simulink model "Fct_app"  (R2018b)
settings: Solver=ode15s  StartTime=0.0  StopTime=T_s  MaxStep=1/(100*fn)  MinStep=1/(1000*fn)  RelTol=1e-3
values from neighbouring files (symbols this model uses):
  f = (alpha/100)*Pn/(Wn)^2    (= 0.000141076783904)    [MAS_EVV_init.m]    (also in fct_trans.m)
  Imr = phi_rd_n/Msr    [MAS_EVV_init.m]    (also in fct_trans.m)
  J = 0.51    [MAS_EVV_init.m]    (also in fct_trans.m)
  k_couple = 1/(0.3*sigma*Ts)    [MAS_EVV_init.m]    (also in fct_trans.m)
  k_omega = 1/(0.3*0.5)    (= 6.66666666667)    [MAS_EVV_init.m]    (also in fct_trans.m)
  k_phi = 1/(0.3*Tr)    [MAS_EVV_init.m]    (also in fct_trans.m)
  Lr = (N2w/2+L1w)/wn    [MAS_EVV_init.m]    (also in fct_trans.m)
  Msr = L1w/wn    [MAS_EVV_init.m]    (also in fct_trans.m)
  P = 1    [MAS_EVV_init.m]    (also in fct_trans.m)
  Rs = 0.9*Rr    [MAS_EVV_init.m]    (also in fct_trans.m)
  sigma = 1-(Msr^2)/(Ls*Lr)    [MAS_EVV_init.m]    (also in fct_trans.m)
  T_C_BF = 0.0445    [MAS_EVV_init.m]    (also in fct_trans.m)
  T_phi_BF = 0.3*Tr    [MAS_EVV_init.m]    (also in fct_trans.m)
  Tr = Lr/Rr    [MAS_EVV_init.m]    (also in fct_trans.m)
  Ts = Ls/Rs    [MAS_EVV_init.m]    (also in fct_trans.m)
  zero_couple = zero(C_couple)    [MAS_EVV_init.m]    (also in fct_trans.m)
  zero_omega = zero(C_omega)    [MAS_EVV_init.m]    (also in fct_trans.m)
  zero_phi = zero(C_phi)    [MAS_EVV_init.m]    (also in fct_trans.m)
undefined symbols (not defined in the file or in its folder): kcouple, komega, kphi
settings Model: Creator=cindyiskandar  LastModifiedBy=cindyiskandar

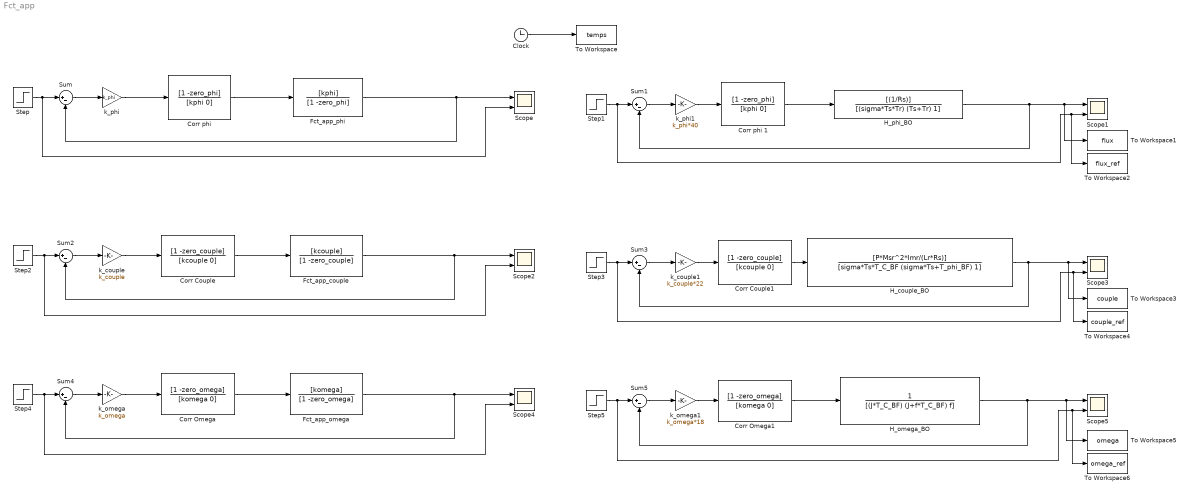
== system Fct_app ==
  Clock : Clock
  Corr Couple : TransferFcn  Numerator=[1 -zero_couple]  Denominator=[kcouple 0]
  Corr Couple1 : TransferFcn  Numerator=[1 -zero_couple]  Denominator=[kcouple 0]
  Corr Omega : TransferFcn  Numerator=[1 -zero_omega]  Denominator=[komega 0]
  Corr Omega1 : TransferFcn  Numerator=[1 -zero_omega]  Denominator=[komega 0]
  "Corr phi " : TransferFcn  Numerator=[1 -zero_phi]  Denominator=[kphi 0]
  Corr phi 1 : TransferFcn  Numerator=[1 -zero_phi]  Denominator=[kphi 0]
  Fct_app_couple : TransferFcn  Numerator=[kcouple]  Denominator=[1 -zero_couple]
  Fct_app_omega : TransferFcn  Numerator=[komega]  Denominator=[1 -zero_omega]
  "Fct_app_phi " : TransferFcn  Numerator=[kphi]  Denominator=[1 -zero_phi]
  H_couple_BO : TransferFcn  Numerator=[P*Msr^2*Imr/(Lr*Rs)]  Denominator=[sigma*Ts*T_C_BF (sigma*Ts+T_phi_BF) 1]
  H_omega_BO : TransferFcn  Denominator=[(J*T_C_BF) (J+f*T_C_BF) f]
  H_phi_BO : TransferFcn  Numerator=[(1/Rs)]  Denominator=[(sigma*Ts*Tr) (Ts+Tr) 1]
  Scope{,1..5} (6 alike) : Scope  NumInputPorts=2
  Step{,1..5} (6 alike) : Step  SampleTime=0
  Sum{,1..5} (6 alike) : Sum  Inputs=|+-
  To Workspace : ToWorkspace  VariableName=temps  SampleTime=-1
      settings: Save2DSignal=2-D array (concatenate along first dimension)
  To Workspace1 : ToWorkspace  VariableName=flux  SampleTime=-1
      settings: Save2DSignal=2-D array (concatenate along first dimension)
  To Workspace2 : ToWorkspace  VariableName=flux_ref  SampleTime=-1
      settings: Save2DSignal=2-D array (concatenate along first dimension)
  To Workspace3 : ToWorkspace  VariableName=couple  SampleTime=-1
      settings: Save2DSignal=2-D array (concatenate along first dimension)
  To Workspace4 : ToWorkspace  VariableName=couple_ref  SampleTime=-1
      settings: Save2DSignal=2-D array (concatenate along first dimension)
  To Workspace5 : ToWorkspace  VariableName=omega  SampleTime=-1
      settings: Save2DSignal=2-D array (concatenate along first dimension)
  To Workspace6 : ToWorkspace  VariableName=omega_ref  SampleTime=-1
      settings: Save2DSignal=2-D array (concatenate along first dimension)
  k_couple : Gain  Gain=k_couple
  k_couple1 : Gain  Gain=k_couple*22
  k_omega : Gain  Gain=k_omega
  k_omega1 : Gain  Gain=k_omega*18
  k_phi : Gain  Gain=k_phi
  k_phi1 : Gain  Gain=k_phi*40
  wires:
  "Corr phi "/1 -> "Fct_app_phi "/1
  k_phi/1 -> "Corr phi "/1
  Step/1 -> Sum/1, Scope/2
  Sum/1 -> k_phi/1
  "Fct_app_phi "/1 -> Sum/2, Scope/1
  k_phi1/1 -> Corr phi 1/1
  Corr phi 1/1 -> H_phi_BO/1
  Sum1/1 -> k_phi1/1
  Step1/1 -> To Workspace2/1, Scope1/2, Sum1/1
  H_phi_BO/1 -> Sum1/2, To Workspace1/1, Scope1/1
  k_couple/1 -> Corr Couple/1
  Corr Couple/1 -> Fct_app_couple/1
  Sum2/1 -> k_couple/1
  Step2/1 -> Scope2/2, Sum2/1
  Fct_app_couple/1 -> Sum2/2, Scope2/1
  k_couple1/1 -> Corr Couple1/1
  Corr Couple1/1 -> H_couple_BO/1
  Sum3/1 -> k_couple1/1
  H_couple_BO/1 -> Sum3/2, To Workspace3/1, Scope3/1
  Step3/1 -> To Workspace4/1, Scope3/2, Sum3/1
  k_omega/1 -> Corr Omega/1
  Corr Omega/1 -> Fct_app_omega/1
  Sum4/1 -> k_omega/1
  Fct_app_omega/1 -> Sum4/2, Scope4/1
  Step4/1 -> Scope4/2, Sum4/1
  Sum5/1 -> k_omega1/1
  Corr Omega1/1 -> H_omega_BO/1
  H_omega_BO/1 -> Sum5/2, To Workspace5/1, Scope5/1
  k_omega1/1 -> Corr Omega1/1
  Step5/1 -> To Workspace6/1, Scope5/2, Sum5/1
  Clock/1 -> To Workspace/1
